simulink model "chap4_7sim"  (Simulink 8.1)
settings: Solver=ode45  StartTime=0.0  StopTime=5  FixedStep=0.001  RelTol=1e-3
settings Model: Creator=ljk  LastModifiedBy=liujk  ExtModeTrigMode=oneshot  ExtModeArmWhenConnect=off
settings DataIOCC: LimitDataPoints=off  SignalLoggingName=sigsOut
settings OptimizationCC: BooleanDataType=off
settings DebuggingCC: SaveWithParameterizedLinksMsg=none  SignalResolutionControl=TryResolveAllWithWarning  SolverPrmCheckMsg=none  MultiTaskDSMMsg=warning  MultiTaskCondExecSysMsg=none  StrictBusMsg=None
settings HardwareCC: TargetUnknown=on
settings RTWCC: IncludeERTFirstTime=on

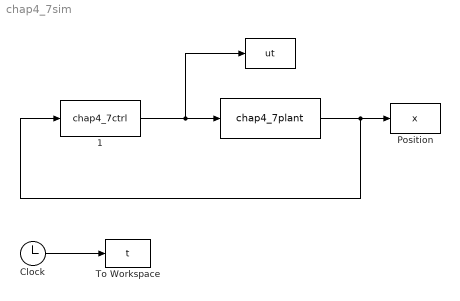
== system chap4_7sim ==
  " " : ToWorkspace  VariableName=ut  SampleTime=-1
  "  " : S-Function  FunctionName=chap4_7plant  EnableBusSupport=off
  "  1" : S-Function  FunctionName=chap4_7ctrl  EnableBusSupport=off
  Clock : Clock
  Position : ToWorkspace  VariableName=x  SampleTime=-1
  To Workspace : ToWorkspace  VariableName=t  SampleTime=-1
  wires:
  "  1"/1 -> "  "/1, " "/1
  "  "/1 -> "  1"/1, Position/1
  Clock/1 -> To Workspace/1
